simulink model "SquatClimbRefinedDesign_new"  (R2025b)
settings: Solver=ode45  StartTime=0.0  StopTime=160  MaxStep=0.002  RelTol=0.01  AbsTol=0.01  EnableMultiTasking=on
undefined symbols (not defined in the file): waypoints, X, Y, Z
libraries: sm_lib x74, nesl_utility x43, slpidlib x2, robotalgslib x1, sharedtransform x1
(part 4 of 4)

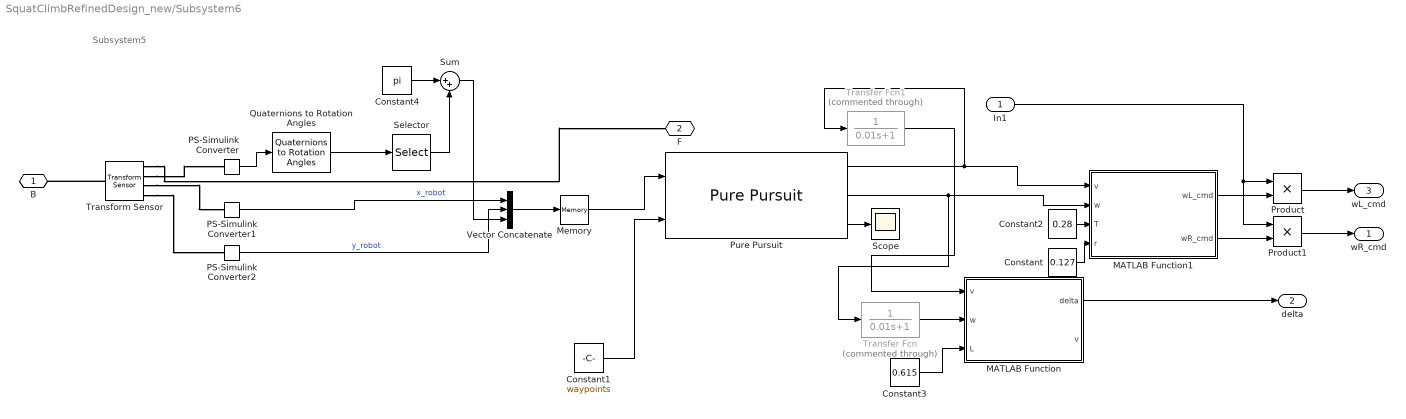
== system SquatClimbRefinedDesign_new/Subsystem6 ==
  note: Subsystem5
  In1 : Inport
  Constant : Constant  Value=0.127
  Constant1 : Constant  Value=waypoints
  Constant2 : Constant  Value=0.28
  Constant3 : Constant  Value=0.615
  Constant4 : Constant  Value=pi
  MATLAB Function : MATLAB Function  TreatAsAtomicUnit=on
  MATLAB Function1 : MATLAB Function  TreatAsAtomicUnit=on
  Memory : Memory
  PS-Simulink Converter : nesl_utility/PS-Simulink Converter  PhysicalDomain=network_engine_domain  SubClassName=ps_output  LeftPortType=input  RightPortType=output  PseudoPeriodic=off  Frequencies=[]  VectorFormat=inherit  Unit=inherit  AffineConversion=off
  PS-Simulink Converter1 : nesl_utility/PS-Simulink Converter  PhysicalDomain=network_engine_domain  SubClassName=ps_output  LeftPortType=input  RightPortType=output  PseudoPeriodic=off  Frequencies=[]  VectorFormat=inherit  Unit=inherit  AffineConversion=off
  PS-Simulink Converter2 : nesl_utility/PS-Simulink Converter  PhysicalDomain=network_engine_domain  SubClassName=ps_output  LeftPortType=input  RightPortType=output  PseudoPeriodic=off  Frequencies=[]  VectorFormat=inherit  Unit=inherit  AffineConversion=off
  Product : Product
  Product1 : Product
  Pure Pursuit : robotalgslib/Pure Pursuit  DesiredLinearVelocityPort=off  DesiredLinearVelocity=0.7  MaxAngularVelocity=0.8  LookaheadDistancePort=off  LookaheadDistance=0.6  TargetDirPort=on  SimulateUsing=Code generation
      settings: LibrarySourceBlock=navlib/Control Algorithms/Pure Pursuit
  Quaternions to Rotation Angles : sharedtransform/Quaternions to Rotation Angles  rotationOrder=ZYX  aMode=aMode
  Scope : Scope
      settings: ActiveDisplayYMinimum=-49.938512022124293  ActiveDisplayYMaximum=229.50278461957694
  Selector : Selector  InputPortWidth=3  IndexOptions=Index vector (dialog)  Indices=[1]  OutputSizes=1
  Sum : Sum  Inputs=|++
  Transfer Fcn : TransferFcn  Commented=through  Denominator=[0.01 1]
  Transfer Fcn1 : TransferFcn  Commented=through  Denominator=[0.01 1]
  Transform Sensor : sm_lib/Frames and Transforms/Transform Sensor  MeasurementFrame=World  RotationSequence=XYX  SenseAngle=off  SenseAxis=off  SenseQ=on  SenseR=off  SenseRotationSequence=off  SenseOmegaX=off  SenseOmegaY=off  SenseOmegaZ=off  SenseOmega=off  SenseQDot=off  SenseRDot=off  SenseRotationSequenceDot=off  SenseAlphaX=off  SenseAlphaY=off  SenseAlphaZ=off  SenseAlpha=off  SenseQDDot=off  SenseRDDot=off  SenseX=on  SenseY=on  SenseZ=off  SenseXYZ=off  SenseRad=off  SenseAzim=off  SenseDist=off  SenseInc=off  SenseXDot=off  SenseYDot=off  SenseZDot=off  SenseXYZDot=off  SenseRadDot=off  SenseAzimDot=off  SenseDistDot=off  SenseIncDot=off  SenseXDDot=off  SenseYDDot=off  SenseZDDot=off  SenseXYZDDot=off  SenseRadDDot=off  SenseAzimDDot=off  SenseDistDDot=off  SenseIncDDot=off
  Vector Concatenate : Concatenate  NumInputs=3
  B : PMIOPort  Side=Right
  F : PMIOPort  Port=2  Side=Right
  wR_cmd : Outport
  delta : Outport  Port=2
  wL_cmd : Outport  Port=3
  wires:
  Pure Pursuit/2 -> MATLAB Function1/2(w), Transfer Fcn/1
  Transfer Fcn1/1 -> MATLAB Function/1("v ")
  Transfer Fcn/1 -> MATLAB Function/2(w)
  Constant1/1 -> Pure Pursuit/2
  Constant/1 -> MATLAB Function1/4(r)
  Constant2/1 -> MATLAB Function1/3(T)
  Constant3/1 -> MATLAB Function/3(L)
  Pure Pursuit/1 -> MATLAB Function1/1(v), Transfer Fcn1/1
  Pure Pursuit/3 -> Scope/1
  Memory/1 -> Pure Pursuit/1
  In1/1 -> Product/1, Product1/1
  MATLAB Function1/1(wL_cmd) -> Product/2
  Product/1 -> wL_cmd/1
  MATLAB Function1/2(wR_cmd) -> Product1/2
  Product1/1 -> wR_cmd/1
  MATLAB Function/1(delta) -> delta/1
  Sum/1 -> Vector Concatenate/3
  Selector/1 -> Sum/2
  Constant4/1 -> Sum/1
  PS-Simulink Converter2/1 -> Vector Concatenate/2  "y_robot"
  PS-Simulink Converter1/1 -> Vector Concatenate/1  "x_robot"
  Vector Concatenate/1 -> Memory/1
  PS-Simulink Converter/1 -> Quaternions to Rotation Angles/1
  Quaternions to Rotation Angles/1 -> Selector/1
  connections:
  Transform Sensor/RConn1 -- F/RConn1
  Transform Sensor/LConn1 -- B/RConn1
  Transform Sensor/RConn3 -- PS-Simulink Converter1/LConn1
  Transform Sensor/RConn2 -- PS-Simulink Converter/LConn1
  Transform Sensor/RConn4 -- PS-Simulink Converter2/LConn1

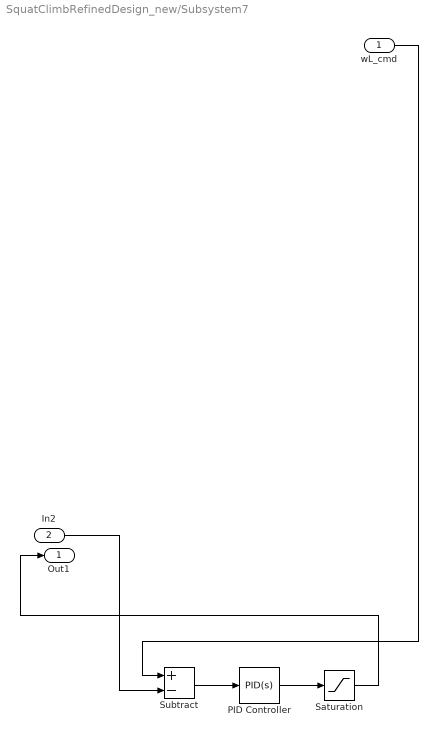
== system SquatClimbRefinedDesign_new/Subsystem7 ==
  wL_cmd : Inport
  In2 : Inport  Port=2
  PID Controller : slpidlib/PID Controller  Controller=PID  Form=Parallel  TimeDomain=Continuous-time  UseExternalTs=off  SampleTime=-1  IntegratorMethod=Forward Euler  FilterMethod=Forward Euler  ControllerParametersSource=internal  P=5  I=0  UseKiTs=off  D=0  UseExternalDerivativeSource=off  N=100  UseFilter=on  TunerSelectOption=Transfer Function Based (PID Tuner App)  InitialConditionSource=internal  InitialConditionForIntegrator=0  InitialConditionForFilter=0  DifferentiatorICPrevScaledInput=0  ExternalReset=none  TrackingMode=off  Kt=1  LimitOutput=off  SatLimitsSource=internal  UpperSaturationLimit=inf  LowerSaturationLimit=-inf  LinearizeAsGain=on  AntiWindupMode=none  Kb=1  LimitIntegrator=off  UpperIntegratorSaturationLimit=inf  LowerIntegratorSaturationLimit=-inf  POutMin=[]  POutMax=[]  IOutMin=[]  IOutMax=[]  DOutMin=[]  DOutMax=[]  NOutMin=[]  NOutMax=[]  SumOutMin=[]  SumOutMax=[]  SaturationOutMin=[]  SaturationOutMax=[]  PParamMin=[]  PParamMax=[]  IParamMin=[]  IParamMax=[]  DParamMin=[]  DParamMax=[]  NParamMin=[]  NParamMax=[]  KbParamMin=[]  KbParamMax=[]  KtParamMin=[]  KtParamMax=[]  KbOutMin=[]  KbOutMax=[]  KtOutMin=[]  KtOutMax=[]  IntegratorOutMin=[]  IntegratorOutMax=[]  FilterOutMin=[]  FilterOutMax=[]  SumI1OutMin=[]  SumI1OutMax=[]  SumI2OutMin=[]  SumI2OutMax=[]  SumI3OutMin=[]  SumI3OutMax=[]  SumI4OutMin=[]  SumI4OutMax=[]  SumDOutMin=[]  SumDOutMax=[]  DifferentiatorOutMin=[]  DifferentiatorOutMax=[]  FilterDiffOutCoefMin=[]  FilterDiffOutCoefMax=[]  ReciprocalOutMin=[]  ReciprocalOutMax=[]  SumDenOutMin=[]  SumDenOutMax=[]  SumNumOutMin=[]  SumNumOutMax=[]  DivideOutMin=[]  DivideOutMax=[]  UdiffTsProdOutMin=[]  UdiffTsProdOutMax=[]  NTsProdOutMin=[]  NTsProdOutMax=[]  UintegralTsProdOutMin=[]  UintegralTsProdOutMax=[]  UngainTsProdOutMin=[]  UngainTsProdOutMax=[]  ClampingZeroOutDataTypeStr=Inherit: Inherit via back propagation  ClampingZeroOutMin=[]  ClampingZeroOutMax=[]  FilterDenConstantOutDataTypeStr=Inherit: Inherit via back propagation  FilterDenConstantOutMin=[]  FilterDenConstantOutMax=[]  PCopyOutDataTypeStr=Inherit: Inherit via back propagation  PCopyOutMin=[]  PCopyOutMax=[]  NCopyOutDataTypeStr=Inherit: Inherit via back propagation  NCopyOutMin=[]  NCopyOutMax=[]  IntegratorContinuousStateAttributes=''  IntegratorStateMustResolveToSignalObject=off  IntegratorRTWStateStorageClass=Auto  FilterContinuousStateAttributes=''  FilterStateMustResolveToSignalObject=off  FilterRTWStateStorageClass=Auto  ParallelPVariant=InternalParameters  IdealPVariant=Disabled  IVariant=InternalParameters  DVariant=InternalParameters  IntegratorVariant=Continuous  SatVariant=Disabled  AWVariant=Passthrough  PCopyVariant=Disabled  TRVariant=Disabled  FdbkBlocksVariant=Forward  IdealPFdbkVariant=Disabled  SatFdbkVariant=Disabled  DerivativeFilterVariant=ContFilter  NVariant=InternalParameters  NCopyVariant=Disabled  FilterICVariant=InternalICsFilter  IntegratorICVariant=InternalICs  ExternalResetVariant=Disabled  TRSumVariant=Passthrough  SumFdbkVariant=Disabled  SumVariant=Sum_PID  TsampFilterVariant=InternalTs  TsampNgainVariant=Passthrough  TsampIntegralVariant=Disabled_SignalSpec  ExternalSaturationOutDataTypeStr=Inherit: Same as second input  DerivativeSourceVariant=ErrorSignal  PreIntVariant=InternalPreInt
  Saturation : Saturate  UpperLimit=5  LowerLimit=-5
  Subtract : Sum  Inputs=+-
  Out1 : Outport
  wires:
  In2/1 -> Subtract/2
  Subtract/1 -> PID Controller/1
  Saturation/1 -> Out1/1
  PID Controller/1 -> Saturation/1
  wL_cmd/1 -> Subtract/1

== matlab function SquatClimbRefinedDesign_new/RL/MATLAB Function1 ==
  data: mode_cmd input; alpha input; tau output; q input; dq input; q_cmd input; is_locked output; q_ref output
function [tau, is_locked, q_ref] = LockJointPD(mode_cmd, alpha, q, dq, q_cmd)
%#codegen
% mode_cmd: 0=Walk (track q_cmd), 1=Wheeled (lock current angle)
% alpha   : [0,1] smoothing factor (TransferFcn output), 0=fully walking, 1=fully locked
% q,dq    : joint angle/angular velocity
% q_cmd   : walk/stand target angle (radians)
Kp = 1200.0;   % Starting value, tune per joint
Kd =   20.0;
tau_lim = 300.0;
m = uint8(mode_cmd ~= 0);     % Standardize to uint8(0/1)
a = double(alpha);
persistent q_hold last_mode
if isempty(q_hold),    q_hold    = q;        end   % double
if isempty(last_mode), last_mode = uint8(0); end   % uint8
% Rising edge: 0->1, latch current angle
if (last_mode == uint8(0)) && (m ~= uint8(0))
    q_hold = q;
end
last_mode = m;
% Reference angle: interpolate between "hold angle" and "target angle"
q_ref  = a*q_hold + (1-a)*q_cmd;
dq_ref = 0.0;
% PD
tau = Kp*(q_ref - q) + Kd*(dq_ref - dq);
% Saturation
tau = max(min(tau, tau_lim), -tau_lim);
% Debug flag: is leg lock dominant
is_locked = (a > 0.5);     % Can also output m==1
end

== matlab function SquatClimbRefinedDesign_new/Subsystem6/MATLAB Function1 ==
  data: v input; wL_cmd output; w input; T input; r input; wR_cmd output
function [wL_cmd, wR_cmd] = wheelSpeedCmd(v, w, T, r)
% v: linear velocity [m/s]
% w: yaw rate [rad/s]
% T: track width [m]
% r: wheel radius [m]

vL = v - 0.5*T*w;
vR = v + 0.5*T*w;

wL_cmd = vL / r;
wR_cmd = vR / r;
end

== matlab function SquatClimbRefinedDesign_new/Subsystem6/MATLAB Function ==
  data: v input; delta output; w input; L input; v output
function [delta, v] = Diff2Ackermann(v, w, L)
% input: 
%   v - Linear velocity (m/s)
%   w - Angular velocity (rad/s)
%   L - Wheelbase (m)
%
% output:
%   delta - front wheel rotation angel (rad)
%   v     -  velocity(m/s)
if abs(v) < 1e-3
    delta = 0;
else
    delta = atan(L * w / v);   % pure pursuit function
end

== matlab function SquatClimbRefinedDesign_new/FR/MATLAB Function2 ==
  data: t input; q_roll output; leg_id input; mode_cmd input
function q_roll = roll_motion_all_legs(t, leg_id, mode_cmd)
    T_walk_start = 130;
    ang_lean = deg2rad(3); 
    smooth_move = @(x) (1 - cos(x*pi))/2;

    if t < T_walk_start
        q_roll = 0; return;
    end

    t_run = t - T_walk_start;
    tau = mod(t_run, 16.0);

    if tau < 2.0; q_roll = smooth_move(tau/2) * (-ang_lean);
    elseif tau < 4.0; q_roll = -ang_lean;
    elseif tau < 6.0; q_roll = -ang_lean + smooth_move((tau-4)/2) * (2*ang_lean);
    elseif tau < 12.0; q_roll = ang_lean;
    elseif tau < 14.0; q_roll = ang_lean + smooth_move((tau-12)/2) * (-2*ang_lean);
    else; q_roll = -ang_lean * (1 - smooth_move((tau-14)/2));
    end
    
end

== matlab function SquatClimbRefinedDesign_new/FL/MATLAB Function2 ==
  data: t input; q_roll output; leg_id input; mode_cmd input
function q_roll = roll_motion_all_legs(t, leg_id, mode_cmd)
    T_walk_start = 130;
    ang_lean = deg2rad(3); 
    smooth_move = @(x) (1 - cos(x*pi))/2;

    if t < T_walk_start
        q_roll = 0; return;
    end

    t_run = t - T_walk_start;
    tau = mod(t_run, 16.0);

   
    if tau < 2.0; q_roll = smooth_move(tau/2) * (-ang_lean);
    elseif tau < 4.0; q_roll = -ang_lean;
    elseif tau < 6.0; q_roll = -ang_lean + smooth_move((tau-4)/2) * (2*ang_lean);
    elseif tau < 12.0; q_roll = ang_lean;
    elseif tau < 14.0; q_roll = ang_lean + smooth_move((tau-12)/2) * (-2*ang_lean);
    else; q_roll = -ang_lean * (1 - smooth_move((tau-14)/2));
    end
    
end

== matlab function SquatClimbRefinedDesign_new/RL/MATLAB Function2 ==
  data: t input; q_roll output; leg_id input; mode_cmd input
function q_roll = roll_motion_all_legs(t, leg_id, mode_cmd)
    T_walk_start = 130;
    ang_lean = deg2rad(3); 
    smooth_move = @(x) (1 - cos(x*pi))/2;

    if t < T_walk_start
        q_roll = 0; return;
    end

    t_run = t - T_walk_start;
    tau = mod(t_run, 16.0);

    if tau < 2.0; q_roll = smooth_move(tau/2) * (-ang_lean);
    elseif tau < 4.0; q_roll = -ang_lean;
    elseif tau < 6.0; q_roll = -ang_lean + smooth_move((tau-4)/2) * (2*ang_lean);
    elseif tau < 12.0; q_roll = ang_lean;
    elseif tau < 14.0; q_roll = ang_lean + smooth_move((tau-12)/2) * (-2*ang_lean);
    else; q_roll = -ang_lean * (1 - smooth_move((tau-14)/2));
    end
    
end

== matlab function SquatClimbRefinedDesign_new/RR/MATLAB Function4 ==
  data: t input; q_roll output; leg_id input; mode_cmd input
function q_roll = roll_motion_all_legs(t, leg_id, mode_cmd)
    T_walk_start = 130;
    ang_lean = deg2rad(3); 
    smooth_move = @(x) (1 - cos(x*pi))/2;

    if t < T_walk_start
        q_roll = 0; return;
    end

    t_run = t - T_walk_start;
    tau = mod(t_run, 16.0);

    
    if tau < 2.0; q_roll = smooth_move(tau/2) * (-ang_lean);
    elseif tau < 4.0; q_roll = -ang_lean;
    elseif tau < 6.0; q_roll = -ang_lean + smooth_move((tau-4)/2) * (2*ang_lean);
    elseif tau < 12.0; q_roll = ang_lean;
    elseif tau < 14.0; q_roll = ang_lean + smooth_move((tau-12)/2) * (-2*ang_lean);
    else; q_roll = -ang_lean * (1 - smooth_move((tau-14)/2));
    end
    
   
end

== matlab function SquatClimbRefinedDesign_new/RR/MATLAB Function1 ==
  data: mode_cmd input; alpha input; tau output; q input; dq input; q_cmd input; is_locked output; q_ref output
function [tau, is_locked, q_ref] = LockJointPD(mode_cmd, alpha, q, dq, q_cmd)
%#codegen
% mode_cmd: 0=Walk (track q_cmd), 1=Wheeled (lock current angle)
% alpha   : [0,1] smoothing factor (TransferFcn output), 0=fully walking, 1=fully locked
% q,dq    : joint angle/angular velocity
% q_cmd   : walk/stand target angle (radians)
Kp = 1200.0;   % Starting value, tune per joint
Kd =   20.0;
tau_lim = 300.0;
m = uint8(mode_cmd ~= 0);     % Standardize to uint8(0/1)
a = double(alpha);
persistent q_hold last_mode
if isempty(q_hold),    q_hold    = q;        end   % double
if isempty(last_mode), last_mode = uint8(0); end   % uint8
% Rising edge: 0->1, latch current angle
if (last_mode == uint8(0)) && (m ~= uint8(0))
    q_hold = q;
end
last_mode = m;
% Reference angle: interpolate between "hold angle" and "target angle"
q_ref  = a*q_hold + (1-a)*q_cmd;
dq_ref = 0.0;
% PD
tau = Kp*(q_ref - q) + Kd*(dq_ref - dq);
% Saturation
tau = max(min(tau, tau_lim), -tau_lim);
% Debug flag: is leg lock dominant
is_locked = (a > 0.5);     % Can also output m==1
end

== matlab function SquatClimbRefinedDesign_new/RL/MATLAB Function3 ==
  data: brake_en input; tau output; w input
function tau = BrakeTorque(brake_en, w)
% brake_en: 0=brake disabled, 1= brake enabled
% w: Wheel angular velocity (rad/s)，output from Revolute Joint Velocity

Kb = 30.0;       % damping coefficient. Higher value=stronger braking
tau_max = 150.0; % maximal braking torque limit
w_eps = 0.05;    % velocity threshold to consider "stopped"

if brake_en == 0
    tau = 0.0;     % brake disabled
    return;
end

% stop applying torque at very low spped to prevent oscillation/jitter
if abs(w) < w_eps
    tau = 0.0;
else
    % damping braking: torque directtion is opposite to angular velocity
    tau = -Kb * w;
end

% torque saturation(limiting)
if tau >  tau_max, tau =  tau_max; end
if tau < -tau_max, tau = -tau_max; end
end

== matlab function SquatClimbRefinedDesign_new/RR/MATLAB Function2 ==
  data: t input; w output
function w = wheel_speed(t)
% WHEEL_SPEED_CONTROLLER 
% This function manages the angular velocity for the rear wheels.
% It executes a sequence of acceleration, constant speed, and braking.
% CRITICAL: At t >= 130s, the wheels are locked (w=0) to support the walking gait.

% ==========================================
% 1. Parameter Definitions
% ==========================================
T_start    = 105;   % Time to begin initial movement (s)
T_accel    = 2;     % Duration of linear acceleration (s)
V_max      = 100;   % Primary target velocity
V_low      = 20;    % Secondary target velocity (used in intermediate phases)

T_dec_init = 125;   % Time to start the first deceleration (s)
T_braking  = 3;     % Duration of the braking phase (s)
T_lock     = 130;   % Global Lock Time: Switch from wheeled to legged mode

% ==========================================
% 2. Logic Control and Phase Switching
% ==========================================

% --- STEP 0: GLOBAL SAFETY LOCK ---
% Once the simulation reaches 130s, the wheels must be strictly locked (0 rad/s).
% This prevents the robot from sliding while the walking gait is active.
if t >= T_lock
    w = 0; 
    return; % Terminate function execution immediately
end

% --- PHASE 1: IDLE / PRE-START ---
% Before T_start, the motor remains stationary.
if t < T_start
    w = 0;

% --- PHASE 2: INITIAL ACCELERATION (0 to V_max) ---
% Linearly ramp up the velocity to minimize mechanical shock.
elseif t < T_start + T_accel
    u = (t - T_start) / T_accel; % Normalized time factor [0 to 1]
    w = u * V_max;

% --- PHASE 3: CONSTANT HIGH-SPEED CRUISE ---
% Maintain V_max for the main wheeled locomotion test.
elseif t < T_dec_init
    w = V_max;

% --- PHASE 4: CONTROLLED DECELERATION (V_max to 0) ---
% Slow down before transitioning to the standing/walking preparation phase.
elseif t < T_dec_init + T_braking
    u = (t - T_dec_init) / T_braking; % Normalized time factor [0 to 1]
    w = V_max * (1 - u);

% --- PHASE 5: PRE-WALK STANDSTILL ---
% Hold the wheel at zero velocity until the T_lock (130s) threshold is met.
else
    w = 0;
end

% Note: Phases previously defined after 130s (e.g., Re-acceleration to V2) 
% have been superseded by the Global Lock at T_lock=130s to ensure 
% the robot remains stable during the walking gait sequence.
end

== matlab function SquatClimbRefinedDesign_new/Front_left_gait/MATLAB Function2 ==
  data: t input; leg_id input; q_hip output; mode_cmd input
function q_hip = hip_motion_all_legs(t, leg_id, mode_cmd)
    T_squat_start = 102;
    T_walk_start  = 130;
    
    if (mode_cmd == 1) || (t < T_squat_start)
        q_hip = 0; return;
    end
    
    % Phase 1: Squat and stand (Note: FR/FL/RR/RL all have a 35-degree spread angle when squatting)
    if t < T_walk_start
        tau = t - T_squat_start;
        q_stand = 0; q_squat = deg2rad(35);
        T1=3; T2=15; T3=3;
        
        if tau < T1; u = tau/T1; q_hip = (1-u)*q_stand + u*q_squat;
        elseif tau < T1+T2; q_hip = q_squat;
        elseif tau < T1+T2+T3; u = (tau-(T1+T2))/T3; q_hip = (1-u)*q_squat + u*q_stand;
        else; q_hip = 0; end
        return;
    end
    
    % Phase 2: Walking logic (Completely retains your Step/Push logic)
    t_run = t - T_walk_start;
    T_cycle = 16.0; tau = mod(t_run, T_cycle);
    ang_step = deg2rad(-10); ang_push = deg2rad(10);
    smooth_move = @(x) (1 - cos(x*pi))/2;
    
    if tau < 4.0 % Phase A
        if tau < 2.0; q_hip = 0; 
        else; s = smooth_move((tau-2)/2);
            if leg_id == 0; q_hip = s * ang_step; else; q_hip = s * ang_push; end
        end
    elseif tau < 8.0 % Phase B
        if tau < 6.0; if leg_id == 0; q_hip = ang_step; else; q_hip = ang_push; end
        else; s = smooth_move((tau-6)/2);
            if leg_id == 2; q_hip = ang_push + s*(ang_step-ang_push);
            elseif leg_id == 0; q_hip = ang_step; else; q_hip = ang_push; end
        end
    elseif tau < 12.0 % Phase C
        if tau < 10.0; if leg_id == 0 || leg_id == 2; q_hip = ang_step; else; q_hip = ang_push; end
        else; s = smooth_move((tau-10)/2);
            if leg_id == 1; q_hip = ang_push + s*(ang_step-ang_push);
            elseif leg_id == 0 || leg_id == 2; q_hip = ang_step; else; q_hip = ang_push; end
        end
    else % Phase D
        if tau < 14.0; if leg_id == 3; q_hip = ang_push; else; q_hip = ang_step; end
        else; s = smooth_move((tau-14)/2);
            if leg_id == 3; q_hip = ang_push + s*(0-ang_push);
            else; q_hip = ang_step + s*(0-ang_step); end
        end
    end
end

== matlab function SquatClimbRefinedDesign_new/FR/MATLAB Function3 ==
  data: t input; torque output; w input
function torque = Front_Wheel_Optimized_Lock(t, w)
% Optimized brake to avoid numerical stiffness
T_lock = 130;
B_heavy = 1000;  % Lowered damping value; 1000 is usually enough to lock a 0.127m wheel
w_threshold = 0.1; % Deadzone threshold (rad/s)

if t < T_lock
    torque = 0;
else
    % Only apply damping when angular velocity exceeds the threshold
    if abs(w) > w_threshold
        torque = -B_heavy * w;
    else
        % At very low speeds, use smaller damping to reduce the burden on the solver
        torque = -B_heavy * 0.1 * w; 
    end
end

== matlab function SquatClimbRefinedDesign_new/Front_left_gait/MATLAB Function3 ==
  data: t input; leg_id input; q_knee output; mode_cmd input
function q_knee = knee_motion_all_legs(t, leg_id, mode_cmd)
    % --- Time Node Definitions ---
    T_squat_start = 102;
    T_walk_start  = 130; 
    
    % Phase 0: Standby
    if (mode_cmd == 1) || (t < T_squat_start)
        q_knee = 0; return;
    end
    
    % Phase 1: Squat and stand (102-130s)
    if t < T_walk_start
        tau = t - T_squat_start;
        q_stand = 0; q_squat = -deg2rad(70);
        T1=3; T2=15; T3=3;
        
        if tau < T1
            u = tau/T1; 
            q_knee = (1-u)*q_stand + u*q_squat;
        elseif tau < T1+T2
            q_knee = q_squat;
        elseif tau < T1+T2+T3
            u = (tau-(T1+T2))/T3; 
            q_knee = (1-u)*q_squat + u*q_stand;
        else
            q_knee = 0; 
        end
        return;
    end
    
    % Phase 2: Walking (130s+)
    t_run = t - T_walk_start;
    T_cycle = 16.0; 
    tau = mod(t_run, T_cycle);
    ang_lift = deg2rad(-12); 
    lift_arch = @(x) sin(x*pi);
    
    q_knee = 0; % Default: no leg lift
    
    if tau >= 2.0 && tau < 4.0 && leg_id == 0 % RF
        q_knee = lift_arch((tau-2)/2) * ang_lift;
    elseif tau >= 6.0 && tau < 8.0 && leg_id == 2 % LR (Note: LR usually denotes Left Rear, but your previous scripts used RL)
        q_knee = lift_arch((tau-6)/2) * ang_lift;
    elseif tau >= 10.0 && tau < 12.0 && leg_id == 1 % LF
        q_knee = lift_arch((tau-10)/2) * ang_lift;
    elseif tau >= 14.0 && tau <= 16.0 && leg_id == 3 % RR
        q_knee = lift_arch((tau-14)/2) * ang_lift;
    end
end

== matlab function SquatClimbRefinedDesign_new/FL/MATLAB Function3 ==
  data: t input; torque output; w input
function torque = Front_Wheel_Optimized_Lock(t, w)
% Optimized brake to avoid numerical stiffness
T_lock = 130;
B_heavy = 1000;  % Lowered damping value; 1000 is usually enough to lock a 0.127m wheel
w_threshold = 0.1; % Deadzone threshold (rad/s)

if t < T_lock
    torque = 0;
else
    % Only apply damping when angular velocity exceeds the threshold
    if abs(w) > w_threshold
        torque = -B_heavy * w;
    else
        % At very low speeds, use smaller damping to reduce the burden on the solver
        torque = -B_heavy * 0.1 * w; 
    end
end

== matlab function SquatClimbRefinedDesign_new/RR/MATLAB Function3 ==
  data: brake_en input; tau output; w input
function tau = BrakeTorque(brake_en, w)
% brake_en: 0=brake disabled, 1= brake enabled
% w: Wheel angular velocity (rad/s)，output from Revolute Joint Velocity

Kb = 30.0;       % damping coefficient. Higher value=stronger braking
tau_max = 150.0; % maximal braking torque limit
w_eps = 0.05;    % velocity threshold to consider "stopped"

if brake_en == 0
    tau = 0.0;     % brake disabled
    return;
end

% stop applying torque at very low spped to prevent oscillation/jitter
if abs(w) < w_eps
    tau = 0.0;
else
    % damping braking: torque directtion is opposite to angular velocity
    tau = -Kb * w;
end

% torque saturation(limiting)
if tau >  tau_max, tau =  tau_max; end
if tau < -tau_max, tau = -tau_max; end
end

== matlab function SquatClimbRefinedDesign_new/Front_right_gait/MATLAB Function1 ==
  data: t input; leg_id input; q_hip output; mode_cmd input
function q_hip = hip_motion_all_legs(t, leg_id, mode_cmd)
    T_squat_start = 102;
    T_walk_start  = 130;
    
    if (mode_cmd == 1) || (t < T_squat_start)
        q_hip = 0; return;
    end
    
    % Phase 1: Squat and stand (Note: FR/FL/RR/RL all have a 35-degree spread angle when squatting)
    if t < T_walk_start
        tau = t - T_squat_start;
        q_stand = 0; q_squat = deg2rad(35);
        T1=3; T2=15; T3=3;
        
        if tau < T1; u = tau/T1; q_hip = (1-u)*q_stand + u*q_squat;
        elseif tau < T1+T2; q_hip = q_squat;
        elseif tau < T1+T2+T3; u = (tau-(T1+T2))/T3; q_hip = (1-u)*q_squat + u*q_stand;
        else; q_hip = 0; end
        return;
    end
    
    % Phase 2: Walking logic (Completely retains your Step/Push logic)
    t_run = t - T_walk_start;
    T_cycle = 16.0; tau = mod(t_run, T_cycle);
    ang_step = deg2rad(-10); ang_push = deg2rad(10);
    smooth_move = @(x) (1 - cos(x*pi))/2;
    
    if tau < 4.0 % Phase A
        if tau < 2.0; q_hip = 0; 
        else; s = smooth_move((tau-2)/2);
            if leg_id == 0; q_hip = s * ang_step; else; q_hip = s * ang_push; end
        end
    elseif tau < 8.0 % Phase B
        if tau < 6.0; if leg_id == 0; q_hip = ang_step; else; q_hip = ang_push; end
        else; s = smooth_move((tau-6)/2);
            if leg_id == 2; q_hip = ang_push + s*(ang_step-ang_push);
            elseif leg_id == 0; q_hip = ang_step; else; q_hip = ang_push; end
        end
    elseif tau < 12.0 % Phase C
        if tau < 10.0; if leg_id == 0 || leg_id == 2; q_hip = ang_step; else; q_hip = ang_push; end
        else; s = smooth_move((tau-10)/2);
            if leg_id == 1; q_hip = ang_push + s*(ang_step-ang_push);
            elseif leg_id == 0 || leg_id == 2; q_hip = ang_step; else; q_hip = ang_push; end
        end
    else % Phase D
        if tau < 14.0; if leg_id == 3; q_hip = ang_push; else; q_hip = ang_step; end
        else; s = smooth_move((tau-14)/2);
            if leg_id == 3; q_hip = ang_push + s*(0-ang_push);
            else; q_hip = ang_step + s*(0-ang_step); end
        end
    end
end

== matlab function SquatClimbRefinedDesign_new/Front_right_gait/MATLAB Function4 ==
  data: t input; leg_id input; q_knee output; mode_cmd input
function q_knee = knee_motion_all_legs(t, leg_id, mode_cmd)
    % --- Time Node Definitions ---
    T_squat_start = 102;
    T_walk_start  = 130; 
    
    % Phase 0: Standby
    if (mode_cmd == 1) || (t < T_squat_start)
        q_knee = 0; return;
    end
    
    % Phase 1: Squat and stand (102-130s)
    if t < T_walk_start
        tau = t - T_squat_start;
        q_stand = 0; q_squat = -deg2rad(70);
        T1=3; T2=15; T3=3;
        
        if tau < T1
            u = tau/T1; 
            q_knee = (1-u)*q_stand + u*q_squat;
        elseif tau < T1+T2
            q_knee = q_squat;
        elseif tau < T1+T2+T3
            u = (tau-(T1+T2))/T3; 
            q_knee = (1-u)*q_squat + u*q_stand;
        else
            q_knee = 0; 
        end
        return;
    end
    
    % Phase 2: Walking (130s+)
    t_run = t - T_walk_start;
    T_cycle = 16.0; 
    tau = mod(t_run, T_cycle);
    ang_lift = deg2rad(-12); 
    lift_arch = @(x) sin(x*pi);
    
    q_knee = 0; % Default: no leg lift
    
    if tau >= 2.0 && tau < 4.0 && leg_id == 0 % RF
        q_knee = lift_arch((tau-2)/2) * ang_lift;
    elseif tau >= 6.0 && tau < 8.0 && leg_id == 2 % LR (Note: LR usually denotes Left Rear, but your previous scripts used RL)
        q_knee = lift_arch((tau-6)/2) * ang_lift;
    elseif tau >= 10.0 && tau < 12.0 && leg_id == 1 % LF
        q_knee = lift_arch((tau-10)/2) * ang_lift;
    elseif tau >= 14.0 && tau <= 16.0 && leg_id == 3 % RR
        q_knee = lift_arch((tau-14)/2) * ang_lift;
    end
end

== matlab function SquatClimbRefinedDesign_new/Rear_right_gait/MATLAB Function2 ==
  data: t input; leg_id input; q_hip output; mode_cmd input
function q_hip = hip_motion_all_legs(t, leg_id, mode_cmd)
    T_squat_start = 102;
    T_walk_start  = 130;
    
    if (mode_cmd == 1) || (t < T_squat_start)
        q_hip = 0; return;
    end
    
    % Phase 1: Squat and stand (Note: FR/FL/RR/RL all have a 35-degree spread angle when squatting)
    if t < T_walk_start
        tau = t - T_squat_start;
        q_stand = 0; q_squat = deg2rad(35);
        T1=3; T2=15; T3=3;
        
        if tau < T1; u = tau/T1; q_hip = (1-u)*q_stand + u*q_squat;
        elseif tau < T1+T2; q_hip = q_squat;
        elseif tau < T1+T2+T3; u = (tau-(T1+T2))/T3; q_hip = (1-u)*q_squat + u*q_stand;
        else; q_hip = 0; end
        return;
    end
    
    % Phase 2: Walking logic (Completely retains your Step/Push logic)
    t_run = t - T_walk_start;
    T_cycle = 16.0; tau = mod(t_run, T_cycle);
    ang_step = deg2rad(-10); ang_push = deg2rad(10);
    smooth_move = @(x) (1 - cos(x*pi))/2;
    
    if tau < 4.0 % Phase A
        if tau < 2.0; q_hip = 0; 
        else; s = smooth_move((tau-2)/2);
            if leg_id == 0; q_hip = s * ang_step; else; q_hip = s * ang_push; end
        end
    elseif tau < 8.0 % Phase B
        if tau < 6.0; if leg_id == 0; q_hip = ang_step; else; q_hip = ang_push; end
        else; s = smooth_move((tau-6)/2);
            if leg_id == 2; q_hip = ang_push + s*(ang_step-ang_push);
            elseif leg_id == 0; q_hip = ang_step; else; q_hip = ang_push; end
        end
    elseif tau < 12.0 % Phase C
        if tau < 10.0; if leg_id == 0 || leg_id == 2; q_hip = ang_step; else; q_hip = ang_push; end
        else; s = smooth_move((tau-10)/2);
            if leg_id == 1; q_hip = ang_push + s*(ang_step-ang_push);
            elseif leg_id == 0 || leg_id == 2; q_hip = ang_step; else; q_hip = ang_push; end
        end
    else % Phase D
        if tau < 14.0; if leg_id == 3; q_hip = ang_push; else; q_hip = ang_step; end
        else; s = smooth_move((tau-14)/2);
            if leg_id == 3; q_hip = ang_push + s*(0-ang_push);
            else; q_hip = ang_step + s*(0-ang_step); end
        end
    end
end

== matlab function SquatClimbRefinedDesign_new/Rear_right_gait/MATLAB Function3 ==
  data: t input; leg_id input; q_knee output; mode_cmd input
function q_knee = knee_motion_all_legs(t, leg_id, mode_cmd)
    % --- Time Node Definitions ---
    T_squat_start = 102;
    T_walk_start  = 130; 
    
    % Phase 0: Standby
    if (mode_cmd == 1) || (t < T_squat_start)
        q_knee = 0; return;
    end
    
    % Phase 1: Squat and stand (102-130s)
    if t < T_walk_start
        tau = t - T_squat_start;
        q_stand = 0; q_squat = -deg2rad(70);
        T1=3; T2=15; T3=3;
        
        if tau < T1
            u = tau/T1; 
            q_knee = (1-u)*q_stand + u*q_squat;
        elseif tau < T1+T2
            q_knee = q_squat;
        elseif tau < T1+T2+T3
            u = (tau-(T1+T2))/T3; 
            q_knee = (1-u)*q_squat + u*q_stand;
        else
            q_knee = 0; 
        end
        return;
    end
    
    % Phase 2: Walking (130s+)
    t_run = t - T_walk_start;
    T_cycle = 16.0; 
    tau = mod(t_run, T_cycle);
    ang_lift = deg2rad(-12); 
    lift_arch = @(x) sin(x*pi);
    
    q_knee = 0; % Default: no leg lift
    
    if tau >= 2.0 && tau < 4.0 && leg_id == 0 % RF
        q_knee = lift_arch((tau-2)/2) * ang_lift;
    elseif tau >= 6.0 && tau < 8.0 && leg_id == 2 % LR (Note: LR usually denotes Left Rear, but your previous scripts used RL)
        q_knee = lift_arch((tau-6)/2) * ang_lift;
    elseif tau >= 10.0 && tau < 12.0 && leg_id == 1 % LF
        q_knee = lift_arch((tau-10)/2) * ang_lift;
    elseif tau >= 14.0 && tau <= 16.0 && leg_id == 3 % RR
        q_knee = lift_arch((tau-14)/2) * ang_lift;
    end
end

== matlab function SquatClimbRefinedDesign_new/Rear_left_gait/MATLAB Function2 ==
  data: t input; leg_id input; q_hip output; mode_cmd input
function q_hip = hip_motion_all_legs(t, leg_id, mode_cmd)
    T_squat_start = 102;
    T_walk_start  = 130;
    
    if (mode_cmd == 1) || (t < T_squat_start)
        q_hip = 0; return;
    end
    
    % Phase 1: Squat and stand (Note: FR/FL/RR/RL all have a 35-degree spread angle when squatting)
    if t < T_walk_start
        tau = t - T_squat_start;
        q_stand = 0; q_squat = deg2rad(35);
        T1=3; T2=15; T3=3;
        
        if tau < T1; u = tau/T1; q_hip = (1-u)*q_stand + u*q_squat;
        elseif tau < T1+T2; q_hip = q_squat;
        elseif tau < T1+T2+T3; u = (tau-(T1+T2))/T3; q_hip = (1-u)*q_squat + u*q_stand;
        else; q_hip = 0; end
        return;
    end
    
    % Phase 2: Walking logic (Completely retains your Step/Push logic)
    t_run = t - T_walk_start;
    T_cycle = 16.0; tau = mod(t_run, T_cycle);
    ang_step = deg2rad(-10); ang_push = deg2rad(10);
    smooth_move = @(x) (1 - cos(x*pi))/2;
    
    if tau < 4.0 % Phase A
        if tau < 2.0; q_hip = 0; 
        else; s = smooth_move((tau-2)/2);
            if leg_id == 0; q_hip = s * ang_step; else; q_hip = s * ang_push; end
        end
    elseif tau < 8.0 % Phase B
        if tau < 6.0; if leg_id == 0; q_hip = ang_step; else; q_hip = ang_push; end
        else; s = smooth_move((tau-6)/2);
            if leg_id == 2; q_hip = ang_push + s*(ang_step-ang_push);
            elseif leg_id == 0; q_hip = ang_step; else; q_hip = ang_push; end
        end
    elseif tau < 12.0 % Phase C
        if tau < 10.0; if leg_id == 0 || leg_id == 2; q_hip = ang_step; else; q_hip = ang_push; end
        else; s = smooth_move((tau-10)/2);
            if leg_id == 1; q_hip = ang_push + s*(ang_step-ang_push);
            elseif leg_id == 0 || leg_id == 2; q_hip = ang_step; else; q_hip = ang_push; end
        end
    else % Phase D
        if tau < 14.0; if leg_id == 3; q_hip = ang_push; else; q_hip = ang_step; end
        else; s = smooth_move((tau-14)/2);
            if leg_id == 3; q_hip = ang_push + s*(0-ang_push);
            else; q_hip = ang_step + s*(0-ang_step); end
        end
    end
end

== matlab function SquatClimbRefinedDesign_new/Rear_left_gait/MATLAB Function4 ==
  data: t input; leg_id input; q_knee output; mode_cmd input
function q_knee = knee_motion_all_legs(t, leg_id, mode_cmd)
    % --- Time Node Definitions ---
    T_squat_start = 102;
    T_walk_start  = 130; 
    
    % Phase 0: Standby
    if (mode_cmd == 1) || (t < T_squat_start)
        q_knee = 0; return;
    end
    
    % Phase 1: Squat and stand (102-130s)
    if t < T_walk_start
        tau = t - T_squat_start;
        q_stand = 0; q_squat = -deg2rad(70);
        T1=3; T2=15; T3=3;
        
        if tau < T1
            u = tau/T1; 
            q_knee = (1-u)*q_stand + u*q_squat;
        elseif tau < T1+T2
            q_knee = q_squat;
        elseif tau < T1+T2+T3
            u = (tau-(T1+T2))/T3; 
            q_knee = (1-u)*q_squat + u*q_stand;
        else
            q_knee = 0; 
        end
        return;
    end
    
    % Phase 2: Walking (130s+)
    t_run = t - T_walk_start;
    T_cycle = 16.0; 
    tau = mod(t_run, T_cycle);
    ang_lift = deg2rad(-12); 
    lift_arch = @(x) sin(x*pi);
    
    q_knee = 0; % Default: no leg lift
    
    if tau >= 2.0 && tau < 4.0 && leg_id == 0 % RF
        q_knee = lift_arch((tau-2)/2) * ang_lift;
    elseif tau >= 6.0 && tau < 8.0 && leg_id == 2 % LR (Note: LR usually denotes Left Rear, but your previous scripts used RL)
        q_knee = lift_arch((tau-6)/2) * ang_lift;
    elseif tau >= 10.0 && tau < 12.0 && leg_id == 1 % LF
        q_knee = lift_arch((tau-10)/2) * ang_lift;
    elseif tau >= 14.0 && tau <= 16.0 && leg_id == 3 % RR
        q_knee = lift_arch((tau-14)/2) * ang_lift;
    end
end

== matlab function SquatClimbRefinedDesign_new/RL/MATLAB Function4 ==
  data: t input; w output
function w = wheel_speed(t)
% WHEEL_SPEED_CONTROLLER 
% This function manages the angular velocity for the rear wheels.
% It executes a sequence of acceleration, constant speed, and braking.
% CRITICAL: At t >= 130s, the wheels are locked (w=0) to support the walking gait.

% ==========================================
% 1. Parameter Definitions
% ==========================================
T_start    = 105;   % Time to begin initial movement (s)
T_accel    = 2;     % Duration of linear acceleration (s)
V_max      = 100;   % Primary target velocity
V_low      = 20;    % Secondary target velocity (used in intermediate phases)

T_dec_init = 125;   % Time to start the first deceleration (s)
T_braking  = 3;     % Duration of the braking phase (s)
T_lock     = 130;   % Global Lock Time: Switch from wheeled to legged mode

% ==========================================
% 2. Logic Control and Phase Switching
% ==========================================

% --- STEP 0: GLOBAL SAFETY LOCK ---
% Once the simulation reaches 130s, the wheels must be strictly locked (0 rad/s).
% This prevents the robot from sliding while the walking gait is active.
if t >= T_lock
    w = 0; 
    return; % Terminate function execution immediately
end

% --- PHASE 1: IDLE / PRE-START ---
% Before T_start, the motor remains stationary.
if t < T_start
    w = 0;

% --- PHASE 2: INITIAL ACCELERATION (0 to V_max) ---
% Linearly ramp up the velocity to minimize mechanical shock.
elseif t < T_start + T_accel
    u = (t - T_start) / T_accel; % Normalized time factor [0 to 1]
    w = u * V_max;

% --- PHASE 3: CONSTANT HIGH-SPEED CRUISE ---
% Maintain V_max for the main wheeled locomotion test.
elseif t < T_dec_init
    w = V_max;

% --- PHASE 4: CONTROLLED DECELERATION (V_max to 0) ---
% Slow down before transitioning to the standing/walking preparation phase.
elseif t < T_dec_init + T_braking
    u = (t - T_dec_init) / T_braking; % Normalized time factor [0 to 1]
    w = V_max * (1 - u);

% --- PHASE 5: PRE-WALK STANDSTILL ---
% Hold the wheel at zero velocity until the T_lock (130s) threshold is met.
else
    w = 0;
end

% Note: Phases previously defined after 130s (e.g., Re-acceleration to V2) 
% have been superseded by the Global Lock at T_lock=130s to ensure 
% the robot remains stable during the walking gait sequence.
end

== matlab function SquatClimbRefinedDesign_new/RR/MATLAB Function ==
  data: mode_cmd input; alpha input; tau output; q input; dq input; q_cmd input; is_locked output; q_ref output
function [tau, is_locked, q_ref] = LockJointPD(mode_cmd, alpha, q, dq, q_cmd)
%#codegen
% mode_cmd: 0=Walk(folloew q_cmd), 1=Wheel(lock the present angle )
% alpha   : [0,1] flatten faktor(TransferFcnoutput)，0=walk, 1=leg locked
% q,dq    : joint angle/angular velocity
% q_cmd   : walking/standing angle(rad)

Kp = 1200.0;   % start value
Kd =   20.0;
tau_lim = 300.0;

m = uint8(mode_cmd ~= 0);     % uint8(0/1)
a = double(alpha);

persistent q_hold last_mode
if isempty(q_hold),    q_hold    = q;        end   % double
if isempty(last_mode), last_mode = uint8(0); end   % uint8

% step: 0->1 
if (last_mode == uint8(0)) && (m ~= uint8(0))
    q_hold = q;
end
last_mode = m;

% reference angle
q_ref  = a*q_hold + (1-a)*q_cmd;
dq_ref = 0.0;

% PD
tau = Kp*(q_ref - q) + Kd*(dq_ref - dq);

% 
tau = max(min(tau, tau_lim), -tau_lim);

% 
is_locked = (a > 0.5);     % 
end

== matlab function SquatClimbRefinedDesign_new/FR/MATLAB Function ==
  data: mode_cmd input; alpha input; tau output; q input; dq input; q_cmd input; is_locked output; q_ref output
function [tau, is_locked, q_ref] = LockJointPD(mode_cmd, alpha, q, dq, q_cmd)
%#codegen
% mode_cmd: 0=Walk (track q_cmd), 1=Wheeled (lock current angle)
% alpha   : [0,1] smoothing factor (TransferFcn output), 0=fully walking, 1=fully locked
% q,dq    : joint angle/angular velocity
% q_cmd   : walk/stand target angle (radians)
Kp = 1200.0;   % Starting value, tune per joint
Kd =   20.0;
tau_lim = 300.0;
m = uint8(mode_cmd ~= 0);     % Standardize to uint8(0/1)
a = double(alpha);
persistent q_hold last_mode
if isempty(q_hold),    q_hold    = q;        end   % double
if isempty(last_mode), last_mode = uint8(0); end   % uint8
% Rising edge: 0->1, latch current angle
if (last_mode == uint8(0)) && (m ~= uint8(0))
    q_hold = q;
end
last_mode = m;
% Reference angle: interpolate between "hold angle" and "target angle"
q_ref  = a*q_hold + (1-a)*q_cmd;
dq_ref = 0.0;
% PD
tau = Kp*(q_ref - q) + Kd*(dq_ref - dq);
% Saturation
tau = max(min(tau, tau_lim), -tau_lim);
% Debug flag: is leg lock dominant
is_locked = (a > 0.5);     % Can also output m==1
end

== matlab function SquatClimbRefinedDesign_new/FR/MATLAB Function1 ==
  data: mode_cmd input; alpha input; tau output; q input; dq input; q_cmd input; is_locked output; q_ref output
function [tau, is_locked, q_ref] = LockJointPD(mode_cmd, alpha, q, dq, q_cmd)
%#codegen
% mode_cmd: 0=Walk (track q_cmd), 1=Wheeled (lock current angle)
% alpha   : [0,1] smoothing factor (TransferFcn output), 0=fully walking, 1=fully locked
% q,dq    : joint angle/angular velocity
% q_cmd   : walk/stand target angle (radians)
Kp = 1200.0;   % Starting value, tune per joint
Kd =   20.0;
tau_lim = 300.0;
m = uint8(mode_cmd ~= 0);     % Standardize to uint8(0/1)
a = double(alpha);
persistent q_hold last_mode
if isempty(q_hold),    q_hold    = q;        end   % double
if isempty(last_mode), last_mode = uint8(0); end   % uint8
% Rising edge: 0->1, latch current angle
if (last_mode == uint8(0)) && (m ~= uint8(0))
    q_hold = q;
end
last_mode = m;
% Reference angle: interpolate between "hold angle" and "target angle"
q_ref  = a*q_hold + (1-a)*q_cmd;
dq_ref = 0.0;
% PD
tau = Kp*(q_ref - q) + Kd*(dq_ref - dq);
% Saturation
tau = max(min(tau, tau_lim), -tau_lim);
% Debug flag: is leg lock dominant
is_locked = (a > 0.5);     % Can also output m==1
end

== matlab function SquatClimbRefinedDesign_new/FL/MATLAB Function ==
  data: mode_cmd input; alpha input; tau output; q input; dq input; q_cmd input; is_locked output; q_ref output
function [tau, is_locked, q_ref] = LockJointPD(mode_cmd, alpha, q, dq, q_cmd)
%#codegen
% mode_cmd: 0=Walk (track q_cmd), 1=Wheeled (lock current angle)
% alpha   : [0,1] smoothing factor (TransferFcn output), 0=fully walking, 1=fully locked
% q,dq    : joint angle/angular velocity
% q_cmd   : walk/stand target angle (radians)
Kp = 1200.0;   % Starting value, tune per joint
Kd =   20.0;
tau_lim = 300.0;
m = uint8(mode_cmd ~= 0);     % Standardize to uint8(0/1)
a = double(alpha);
persistent q_hold last_mode
if isempty(q_hold),    q_hold    = q;        end   % double
if isempty(last_mode), last_mode = uint8(0); end   % uint8
% Rising edge: 0->1, latch current angle
if (last_mode == uint8(0)) && (m ~= uint8(0))
    q_hold = q;
end
last_mode = m;
% Reference angle: interpolate between "hold angle" and "target angle"
q_ref  = a*q_hold + (1-a)*q_cmd;
dq_ref = 0.0;
% PD
tau = Kp*(q_ref - q) + Kd*(dq_ref - dq);
% Saturation
tau = max(min(tau, tau_lim), -tau_lim);
% Debug flag: is leg lock dominant
is_locked = (a > 0.5);     % Can also output m==1
end

== matlab function SquatClimbRefinedDesign_new/FL/MATLAB Function1 ==
  data: mode_cmd input; alpha input; tau output; q input; dq input; q_cmd input; is_locked output; q_ref output
function [tau, is_locked, q_ref] = LockJointPD(mode_cmd, alpha, q, dq, q_cmd)
%#codegen
% mode_cmd: 0=Walk (track q_cmd), 1=Wheeled (lock current angle)
% alpha   : [0,1] smoothing factor (TransferFcn output), 0=fully walking, 1=fully locked
% q,dq    : joint angle/angular velocity
% q_cmd   : walk/stand target angle (radians)
Kp = 1200.0;   % Starting value, tune per joint
Kd =   20.0;
tau_lim = 300.0;
m = uint8(mode_cmd ~= 0);     % Standardize to uint8(0/1)
a = double(alpha);
persistent q_hold last_mode
if isempty(q_hold),    q_hold    = q;        end   % double
if isempty(last_mode), last_mode = uint8(0); end   % uint8
% Rising edge: 0->1, latch current angle
if (last_mode == uint8(0)) && (m ~= uint8(0))
    q_hold = q;
end
last_mode = m;
% Reference angle: interpolate between "hold angle" and "target angle"
q_ref  = a*q_hold + (1-a)*q_cmd;
dq_ref = 0.0;
% PD
tau = Kp*(q_ref - q) + Kd*(dq_ref - dq);
% Saturation
tau = max(min(tau, tau_lim), -tau_lim);
% Debug flag: is leg lock dominant
is_locked = (a > 0.5);     % Can also output m==1
end

== matlab function SquatClimbRefinedDesign_new/RL/MATLAB Function ==
  data: mode_cmd input; alpha input; tau output; q input; dq input; q_cmd input; is_locked output; q_ref output
function [tau, is_locked, q_ref] = LockJointPD(mode_cmd, alpha, q, dq, q_cmd)
%#codegen
% mode_cmd: 0=Walk (track q_cmd), 1=Wheeled (lock current angle)
% alpha   : [0,1] smoothing factor (TransferFcn output), 0=fully walking, 1=fully locked
% q,dq    : joint angle/angular velocity
% q_cmd   : walk/stand target angle (radians)
Kp = 1200.0;   % Starting value, tune per joint
Kd =   20.0;
tau_lim = 300.0;
m = uint8(mode_cmd ~= 0);     % Standardize to uint8(0/1)
a = double(alpha);
persistent q_hold last_mode
if isempty(q_hold),    q_hold    = q;        end   % double
if isempty(last_mode), last_mode = uint8(0); end   % uint8
% Rising edge: 0->1, latch current angle
if (last_mode == uint8(0)) && (m ~= uint8(0))
    q_hold = q;
end
last_mode = m;
% Reference angle: interpolate between "hold angle" and "target angle"
q_ref  = a*q_hold + (1-a)*q_cmd;
dq_ref = 0.0;
% PD
tau = Kp*(q_ref - q) + Kd*(dq_ref - dq);
% Saturation
tau = max(min(tau, tau_lim), -tau_lim);
% Debug flag: is leg lock dominant
is_locked = (a > 0.5);     % Can also output m==1
end
